simulink model "Sottrazione_Spettrale"  (R2020a)
settings: Solver=VariableStepAuto  StartTime=0.0  StopTime=20.0  RelTol=1e-3
libraries: dspxfrm3 x3, dspsigops x2, dspsnks4 x1, simulink x1, dspvision x1, dspstat3 x1
settings Model: Creator=Michele  LastModifiedBy=miche
settings DataIOCC: ReturnWorkspaceOutputs=off
settings DebuggingCC: ArithmeticOperatorsInVariantConditions=warning
settings SFSimCC: SimUseLocalCustomCode=off  CustomCodeUndefinedFunction=UseInterfaceOnly
settings RTWCC: RTWUseLocalCustomCode=off
settings CodeAppCC: StateflowObjectComments=on

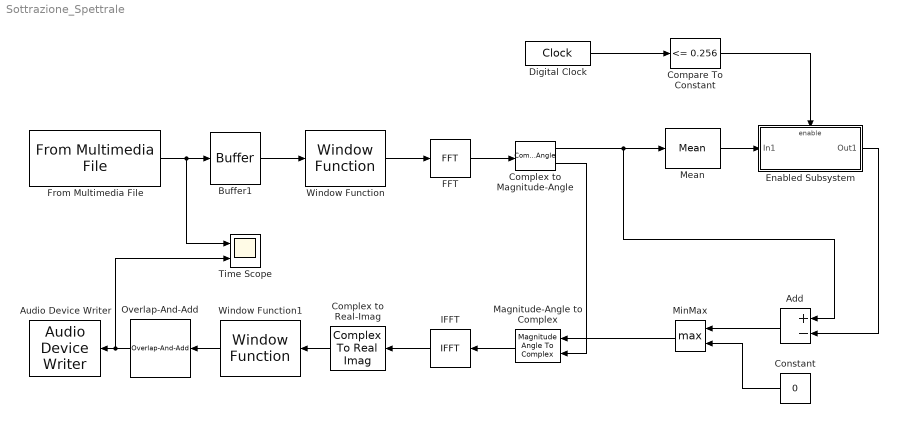
== system Sottrazione_Spettrale ==
  Add : Sum  Inputs=+-
  Audio Device Writer : dspsnks4/Audio Device Writer  Driver=DirectSound  Device=Default  InheritSampleRate=on  SampleRate=44100  BitDepth=16-bit integer  BufferSize=4096  NumBuffers=10  DefaultOutputChannelMapping=on  OutputChannelMapping=1:2  OutputNumUnderrunSamples=off  DriverIdx=1  DeviceWarnFlag=''
  Buffer1 : Buffer  N=512  V=256  OutputFrames=off
  Compare To Constant : simulink/Logic and Bit Operations/Compare To Constant  relop=<=  const=0.256  OutDataTypeStr=boolean
  Complex to Magnitude-Angle : ComplexToMagnitudeAngle
  Complex to Real-Imag : ComplexToRealImag  Output=Real
  Constant : Constant  Value=0
  Digital Clock : DigitalClock  SampleTime=512/8000
  Enabled Subsystem : Subsystem  TreatAsAtomicUnit=on
  FFT : dspxfrm3/FFT  FFTImplementation=Auto  CompMethod=Table lookup  TableOpt=NEW  TableOptActive=Speed  BitRevOrder=off  Normalize=off  InheritFFTLength=on  FFTLength=64  WrapInput=on  roundingMode=Floor  overflowMode=off  firstCoeffDataTypeStr=Inherit: Same word length as input  firstCoeffLastDataTypeStr=Inherit: Same word length as input  outputMin=[]  outputMax=[]
  From Multimedia File : dspvision/From Multimedia File  inputFilename=C:\Users\miche\Documents\MATLAB\radio_noise.wav  readRange=[1 Inf]  loop=on  numPlays=inf  outputStreams=Audio only  videoDataType=single  audioDataType=double  inheritSampleTime=on  userDefinedSampleTime=1/30  noAudioOutput=off  isIntensityVideo=off  fourcc=RGB  colorVideoFormat=Separate color signals  outputEOF=off  dataOrg=Column-major  audioFrameSize=512  computeAudioFrameSize=off  outSamplingMode=Sample based
  IFFT : dspxfrm3/IFFT  FFTImplementation=Auto  CompMethod=Table lookup  TableOpt=NEW  TableOptActive=Speed  BitRevOrder=off  cs_in=off  Normalize=on  InheritFFTLength=on  FFTLength=64  WrapInput=on  mode=Complex  outSamplingMode=Sample based  roundingMode=Floor  overflowMode=off  firstCoeffDataTypeStr=Inherit: Same word length as input  firstCoeffLastDataTypeStr=Inherit: Same word length as input  outputMin=[]  outputMax=[]
  Magnitude-Angle to Complex : MagnitudeAngleToComplex
  Mean : dspstat3/Mean  run=off  InputProcessing=Columns as channels (frame based)  reset_popup=None  directionMode=Each column  dimension=1  roiEnable=off  roiType=Rectangles  roiPortion=Entire ROI  roiOutput=Individual statistics for each ROI  roiFlag=off  roundingMode=Floor  overflowMode=off  outputDataTypeStr=Inherit: Same as accumulator  outputMin=[]  outputMax=[]  outputLastDataTypeStr=Inherit: Same as accumulator
  MinMax : MinMax  Function=max  Inputs=2
  Overlap-And-Add : dspxfrm3/Inverse  Short-Time FFT/Overlap-And-Add  L=256
      settings: SourceProductBaseCode=DS
  Time Scope : Scope  NumInputPorts=2
  Window Function : dspsigops/Window Function  winmode=Apply window to input  wintype=Hanning  sampmode=Continuous  samptime=1  N=64  Rs=50  beta=10  winsamp=Periodic  UserWindow=hamming  OptParams=off  UserParams={'symmetric'}  dataType=double  isSigned=on  wordLen=16  udDataType=sfix(16)  fracBitsMode=Best precision  numFracBits=15  roundingMode=Floor  overflowMode=off  numSidelobes=4  sidelobeLevel=-30
      settings: SourceProductBaseCode=DS
  Window Function1 : dspsigops/Window Function  winmode=Apply window to input  wintype=Hanning  sampmode=Continuous  samptime=1  N=64  Rs=50  beta=10  winsamp=Periodic  UserWindow=hamming  OptParams=off  UserParams={'symmetric'}  dataType=double  isSigned=on  wordLen=16  udDataType=sfix(16)  fracBitsMode=Best precision  numFracBits=15  roundingMode=Floor  overflowMode=off  numSidelobes=4  sidelobeLevel=-30
      settings: SourceProductBaseCode=DS
  wires:
  FFT/1 -> Complex to Magnitude-Angle/1
  Complex to Real-Imag/1 -> Window Function1/1
  Magnitude-Angle to Complex/1 -> IFFT/1
  Add/1 -> MinMax/1
  Complex to Magnitude-Angle/2 -> Magnitude-Angle to Complex/2
  IFFT/1 -> Complex to Real-Imag/1
  Constant/1 -> MinMax/2
  Digital Clock/1 -> Compare To Constant/1
  Compare To Constant/1 -> Enabled Subsystem/Enable
  From Multimedia File/1 -> Time Scope/1, Buffer1/1
  Mean/1 -> Enabled Subsystem/1(In1)
  Buffer1/1 -> Window Function/1
  Overlap-And-Add/1 -> Time Scope/2, Audio Device Writer/1
  Window Function/1 -> FFT/1
  Window Function1/1 -> Overlap-And-Add/1
  Complex to Magnitude-Angle/1 -> Add/1, Mean/1
  MinMax/1 -> Magnitude-Angle to Complex/1
  Enabled Subsystem/1(Out1) -> Add/2

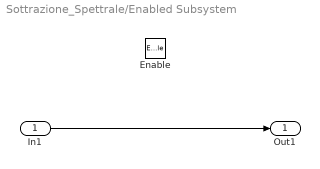
== system Sottrazione_Spettrale/Enabled Subsystem ==
  In1 : Inport
  Enable : EnablePort
  Out1 : Outport
  wires:
  In1/1 -> Out1/1
